simulink model "Linearization2"  (R2022a)
settings: Solver=VariableStepAuto  StartTime=0.0  StopTime=10.0  RelTol=1e-3
undefined symbols (not defined in the file): Aactuator, ac, AeroCoeff, ControlAllocation, DUmax, DUmin, EngineTable, F, fcs, ft, g, hground, IC, kg, LandingGear, Light, LPmethod, m, MIL, Mode_deflection_aileron, Mode_deflection_elevator, Mode_deflection_rudder, Mode_deflection_TVC_y, Mode_deflection_TVC_z, N, Ninv_2nozzle, Ninv_no_nozzle, PIController, s, Sensor, slug, state0, sysID_DAQ, sysID_OBES, Umax_2nozzle, Umax_no_nozzle, Umin_2nozzle, Umin_no_nozzle, WMM2020
libraries: aerolibconvert2 x19, slpidlib x6, simulink x6, sharedutil x4, aerolibatmos2 x3, aerolibwind2 x3, aerolibbdyn x3, aerolibgravity2 x2, sharedtransform x1
(part 2 of 9)

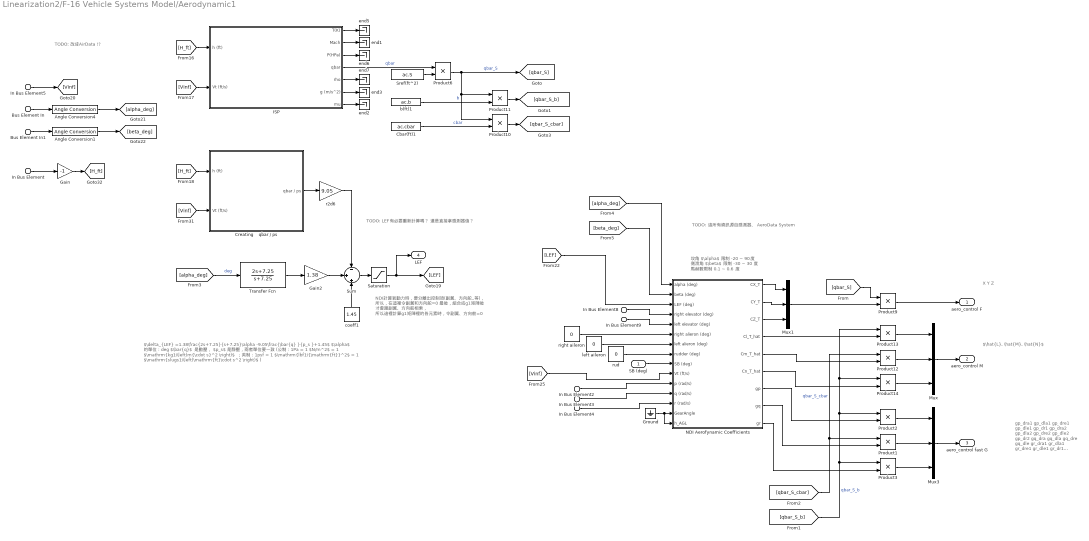
== system Linearization2/F-16 Vehicle Systems Model/Aerodynamic1 ==
  note: NDI計算氣動力時，要分離出控制項(副翼、方向舵..等)，
      | 所以，在這裡令副翼和方向舵=0
      | 最後，組合成g1矩陣後 才會跟副翼、方向舵相乘，
      | 所以這裡計算g1矩陣裡的各元素時，令副翼、方向舵=0
  note: TODO: LEF有必要重新計算嗎？
      | 還是直接拿感測器值？
  note: X
      | Y
      | Z
  note: $\delta_{LEF} =1.38\frac{2s+7.25}{s+7.25}\alpha -9.05\frac{\bar{q} }{p_s }+1.45$
      | $\alpha$ 的單位：deg
      | $\bar{q}$ 是動壓， $p_s$ 是靜壓，兩者單位要一致 (公制：1Pa = 1 $N/m^2$ = 1 $\mathrm{kg}/\left(m{\cdot s}^2 \right)$ ；英制：1psf = 1 $\mathrm{lbf}/{\mathrm{ft}}^2$ = 1 $\mathrm{slugs}/\left(\mathrm{ft}\cdot s^2 \right)$ )
  note: $\hat{L}, \hat{M}, \hat{N}$
  note: TODO: 這所有資訊源自感測器、
      | AeroData System
  note: TODO: 改成AirData !?
  note: 攻角 $\alpha$ 限制 -20 ~ 90度
      | 側滑角 $\beta$ 限制 -30 ~ 30 度
      | 馬赫數限制 0.1 ~ 0.6 度
  note: gp_dra1
      | gp_dla1
      | gp_dre1
      | gp_dle1
      | gp_dr1
      | gp_dra2
      | gp_dla2
      | gp_dre2
      | gp_dle2
      | gp_dr2
      |
      | gq_dra
      | gq_dla
      | gq_dre
      | gq_dle
      |
      | gr_dra1
      | gr_dla1
      | gr_dre1
      | gr_dle1
      | gr_dr1
      | gr_dra2
      | gr_dla2
      | gr_dre2
      | gr_dle2
      | gr_dr2
  SB (deg) : Inport  Unit=deg
  In Bus Element : Inport  Port=2  PortName=PlantData  Element=altitude
  In Bus Element8 : Inport  Port=2  PortName=PlantData  Element=AeroActBus.right Elevator_deg
  In Bus Element9 : Inport  Port=2  PortName=PlantData  Element=AeroActBus.left Elevator_deg
  In Bus Element2 : Inport  Port=2  PortName=PlantData  Element=p
  In Bus Element3 : Inport  Port=2  PortName=PlantData  Element=q
  In Bus Element4 : Inport  Port=2  PortName=PlantData  Element=r
  In Bus Element5 : Inport  Port=2  PortName=PlantData  Element=Vt
  Bus Element In : Inport  Port=3  PortName=AirData  Element=alpha
  Bus Element In1 : Inport  Port=3  PortName=AirData  Element=beta
  Angle Conversion1 : aerolibconvert2/Angle Conversion  IU=rad  OU=deg
  Angle Conversion4 : aerolibconvert2/Angle Conversion  IU=rad  OU=deg
  Cbar(ft)1 : Constant  Value=ac.cbar
  Creating    qbar / ps : Subsystem
  Gain : Gain  Gain=-1
  Gain2 : Gain  Gain=1.38  SaturateOnIntegerOverflow=on  OutDataTypeStr=Inherit: Same as input  ParamDataTypeStr=Inherit: Same as input
  Ground : Ground
  "ISP " : Subsystem
  Mux : Mux  Inputs=3
  Mux1 : Mux  Inputs=3
  Mux3 : Mux  Inputs=3
  NDI Aerofynamic Coefficients : Subsystem
  Product{1..3,6,9..14} (10 alike) : Product
  Saturation : Saturate  UpperLimit=Aactuator.LEF.AngleLimitUpper  LowerLimit=Aactuator.LEF.AngleLimitLower
  Sref(ft^2) : Constant  Value=ac.S
  Sum : Sum  Inputs=-|+|+  InputSameDT=on  SaturateOnIntegerOverflow=on  OutDataTypeStr=Inherit: Same as first input
  Transfer Fcn : TransferFcn  Numerator=[2 7.25]  Denominator=[1 7.25]
  b(ft)1 : Constant  Value=ac.b
  coeff1 : Constant  Value=1.45
  end{1..3,5..7} (6 alike) : Terminator
  left aileron : Constant  Value=0
  r2d6 : Gain  Gain=9.05  SaturateOnIntegerOverflow=on  OutDataTypeStr=Inherit: Same as input  ParamDataTypeStr=Inherit: Same as input
  right aileron : Constant  Value=0
  rud : Constant  Value=0
  aero_control F : Outport  VectorParamsAs1DForOutWhenUnconnected=off
  aero_control M : Outport  Port=2  VectorParamsAs1DForOutWhenUnconnected=off
  aero_control fast G : Outport  Port=3  VectorParamsAs1DForOutWhenUnconnected=off
  LEF : Outport  Port=4
  wires:
  [Vinf] -> "ISP "/2(Vt (ft/s))
  "ISP "/2("Mach ") -> end1/1
  "ISP "/7(mu) -> end2/1
  "ISP "/6(g (m/s^2)) -> end3/1
  "ISP "/5(rho) -> end7/1
  "ISP "/4("qbar ") -> Product6/1  "qbar"
  "ISP "/3(P(HPa)) -> end6/1
  "ISP "/1(T(K)) -> end5/1
  r2d6/1 -> Sum/1
  Creating    qbar / ps/1(qbar / ps) -> r2d6/1
  [alpha_deg] -> Transfer Fcn/1  "deg"
  [Vinf] -> Creating    qbar / ps/2(Vt (ft/s))
  coeff1/1 -> Sum/3
  [H_ft] -> Creating    qbar / ps/1(h (ft))
  [H_ft] -> "ISP "/1(h (ft))
  Sum/1 -> Saturation/1
  Saturation/1 -> LEF/1, [LEF]
  Transfer Fcn/1 -> Gain2/1
  In Bus Element/1 -> Gain/1
  Gain/1 -> [H_ft]
  Cbar(ft)1/1 -> Product10/2  "cbar"
  b(ft)1/1 -> Product11/2  "b"
  Sref(ft^2)/1 -> Product6/2
  Product10/1 -> [qbar_S_cbar]
  Product6/1 -> Product11/1, Product10/1, [qbar_S]  "qbar_S"
  Product11/1 -> [qbar_S_b]
  [qbar_S] -> Product9/1
  Product9/1 -> aero_control F/1
  Product12/1 -> Mux/2
  Product13/1 -> Mux/1
  Product14/1 -> Mux/3
  Mux/1 -> aero_control M/1
  NDI Aerofynamic Coefficients/4(Cl_T_hat) -> Product13/2
  NDI Aerofynamic Coefficients/5(Cm_T_hat) -> Product12/2
  NDI Aerofynamic Coefficients/6(Cn_T_hat) -> Product14/2
  NDI Aerofynamic Coefficients/1(CX_T) -> Mux1/1
  NDI Aerofynamic Coefficients/2(CY_T) -> Mux1/2
  NDI Aerofynamic Coefficients/3(CZ_T) -> Mux1/3
  Mux1/1 -> Product9/2
  [qbar_S_b] -> Product13/1, Product14/1, Product2/1, Product3/1  "qbar_S_b"
  Product3/1 -> Mux3/3
  Product1/1 -> Mux3/2
  Product2/1 -> Mux3/1
  NDI Aerofynamic Coefficients/7(gp) -> Product2/2
  [qbar_S_cbar] -> Product12/1, Product1/1  "qbar_S_cbar"
  NDI Aerofynamic Coefficients/9(gr) -> Product3/2
  NDI Aerofynamic Coefficients/8(gq) -> Product1/2
  Mux3/1 -> aero_control fast G/1
  [Vinf] -> NDI Aerofynamic Coefficients/10(Vt (ft/s))
  SB (deg)/1 -> NDI Aerofynamic Coefficients/9(SB (deg))
  [LEF] -> NDI Aerofynamic Coefficients/3(LEF (deg))
  [beta_deg] -> NDI Aerofynamic Coefficients/2(beta (deg))
  [alpha_deg] -> NDI Aerofynamic Coefficients/1(alpha (deg))
  In Bus Element2/1 -> NDI Aerofynamic Coefficients/11(p (rad/s))
  In Bus Element3/1 -> NDI Aerofynamic Coefficients/12(q (rad/s))
  In Bus Element4/1 -> NDI Aerofynamic Coefficients/13(r (rad/s))
  Ground/1 -> NDI Aerofynamic Coefficients/14(GearAngle), NDI Aerofynamic Coefficients/15(h_AGL)
  Gain2/1 -> Sum/2
  Bus Element In/1 -> Angle Conversion4/1
  Angle Conversion4/1 -> [alpha_deg]
  Angle Conversion1/1 -> [beta_deg]
  Bus Element In1/1 -> Angle Conversion1/1
  In Bus Element5/1 -> [Vinf]
  In Bus Element8/1 -> NDI Aerofynamic Coefficients/4(right elevator (deg))
  In Bus Element9/1 -> NDI Aerofynamic Coefficients/5(left elevator (deg))
  right aileron/1 -> NDI Aerofynamic Coefficients/6(right alieron (deg))
  left aileron/1 -> NDI Aerofynamic Coefficients/7(left alieron (deg))
  rud/1 -> NDI Aerofynamic Coefficients/8(rudder (deg))

== system Linearization2/F-16 Vehicle Systems Model/Rotation Speed(TVC OFF)OK ==
  pqr command : Inport
  In Bus Element : Inport  Port=2  PortName=PlantData  Element=Vt
  Constant : Constant  Value=0
  If : If  IfExpression=u1 > 220  ElseIfExpressions=220 >= u1 >= 135
  If Action Subsystem : Subsystem  TreatAsAtomicUnit=on
  If Action Subsystem1 : Subsystem  TreatAsAtomicUnit=on
  Merge : Merge
  Terminator1 : Terminator
  Output : Outport
  wires:
  If/1 -> If Action Subsystem/Action
  Constant/1 -> If Action Subsystem1/1(In1)
  If Action Subsystem1/1(Out1) -> Merge/2
  If Action Subsystem/1(Out1) -> Merge/1
  pqr command/1 -> If Action Subsystem/1(pqr command)
  Merge/1 -> Output/1
  In Bus Element/1 -> If/1
  If/2 -> If Action Subsystem1/Action
  If/3 -> Terminator1/1

== system Linearization2/F-16 Vehicle Systems Model/Vehicle ==
  note: 重心高度只取體軸z，因假設機腹朝下。
      | 更正確做法是要乘上旋轉座標DCM_eb
  note: 為了避免無謂計算，縮短模擬時間，
      | 只有在「飛機重心靠近地面」並且「起落架放下」的情況，
      | 才開始計算地面反作用力
  note: 設定Port dimensions=3
  note: 攻角 $\alpha$ 限制 -20 ~ 90度
      | 側滑角 $\beta$ 限制 -30 ~ 30 度
      | 馬赫數限制 0.1 ~ 0.6 度
  note: Tx
      | Ty
      | Tz
      | ---
      | Mx_T
      | My_T
      | Mz_T
  note: 高度限制 0 ~ 50000 ft
      | 馬赫數限制 0 ~ 1 馬赫
  note: f
      | 0
      | N
  note: TODO: 改成local變數
      | 或者應該新增為OBM機載模型!?
      | 或者空中NDI跟地面NDI控制器分離!?
  note: Nonlinear Model
  fadec_cmd : Inport
  fcs_cmd : Inport  Port=2
  " SB_deg" : Inport  Port=3
  LG_cmd : Inport  Port=4
  Bus Element In{,1..3} (4 alike) : Inport  Port=5  PortName=EnvData
  In Bus Element : Inport  Port=5  PortName=EnvData  Element=g
  LogDataBus : Inport  Port=6
  6DOF (Quaternion) : Subsystem
  Actuators (no roll off)1 : Subsystem  Commented=on
  Aerodynamics : Subsystem
  Bus Selector : BusSelector  OutputSignals=altitude
  Compare To Constant : simulink/Logic and Bit Operations/Compare To Constant  relop=>=  const=-30  OutDataTypeStr=boolean
  Demux2 : Demux  Outputs=[3, 3]
  Demux3 : Demux  Outputs=3
  Demux4 : Demux  Outputs=[3, 3]
  Gravity Force : Subsystem
  LandingGear GroundReaction : Subsystem
  Logical Operator : Logic  AllPortsSameDT=off  OutDataTypeStr=boolean
  Logical Operator1 : Logic  Operator=OR  Inputs=1  AllPortsSameDT=off  OutDataTypeStr=boolean
  ModelBus : BusCreator  Inputs=39
  Propulsion : Subsystem  Commented=on
  Propulsion(two_nozzles) : Subsystem
  Selector : Selector  InputPortWidth=3  IndexOptions=Index vector (dialog)  Indices=3  OutputSizes=1
  Selector1 : Selector  InputPortWidth=6  IndexOptions=Index vector (dialog)  Indices=[1 2 3]  OutputSizes=1
  Selector2 : Selector  InputPortWidth=6  IndexOptions=Index vector (dialog)  Indices=[1 2 3]  OutputSizes=1
  Signal Specification : SignalSpecification  Dimensions=3
  Sum : Sum  Inputs=||+++
  Sum1 : Sum  Inputs=++|
  Terminator3 : Terminator
  PlantData : Outport
  tag scope: LGxyz=global
  wires:
  " SB_deg"/1 -> Aerodynamics/2(" SB (deg)")
  Aerodynamics/1(FM) -> Sum/2, 6DOF (Quaternion)/4(AeroFM)
  Aerodynamics/2(ActSensor_Out) -> [AeroActBus]
  Propulsion(two_nozzles)/1(FM) -> Selector2/1, Sum/1
  fcs_cmd/1 -> Aerodynamics/1(fcs_cmd), [fcs_cmd]  "fcs_cmd"
  fadec_cmd/1 -> Propulsion(two_nozzles)/1(fadec_cmd), [fadec_cmd]  "fadec_cmd"
  Propulsion(two_nozzles)/2(ActSensor_Out) -> [PropActBus]
  Propulsion(two_nozzles)/3(PropData) -> [PropBus]
  Sum/1 -> Demux4/1
  Sum1/1 -> 6DOF (Quaternion)/1(Fxyz)
  Bus Element In/1 -> Aerodynamics/3(EnvData)
  Bus Element In1/1 -> Propulsion(two_nozzles)/2(EnvData)
  LandingGear GroundReaction/1(FM) -> Demux2/1, Sum/3, Selector1/1
  Selector1/1 -> 6DOF (Quaternion)/5(LGxyz)
  Demux2/1 -> [LGxyz]
  Demux2/2 -> Terminator3/1
  Signal Specification/1 -> Logical Operator1/1, LandingGear GroundReaction/1(LG_cmd)
  LandingGear GroundReaction/2(LGData) -> [LGBus]
  Logical Operator/1 -> LandingGear GroundReaction/Enable
  Compare To Constant/1 -> Logical Operator/1
  Bus Selector/1 -> Compare To Constant/1  "<altitude>"
  Logical Operator1/1 -> Logical Operator/2
  LG_cmd/1 -> Signal Specification/1
  Gravity Force/1(Fgrav) -> Sum1/1
  Demux4/1 -> Sum1/2
  Bus Element In3/1 -> Gravity Force/2(EnvData)
  Bus Element In2/1 -> LandingGear GroundReaction/2(EnvData)
  In Bus Element/1 -> Selector/1
  [PropActBus] -> ModelBus/35  "PropActBus"
  Demux3/2 -> ModelBus/31
  6DOF (Quaternion)/22(ay_cg) -> ModelBus/22  "ay_cg"
  Demux3/3 -> ModelBus/32  "N"
  Demux3/1 -> ModelBus/30  "f"
  6DOF (Quaternion)/2(DCM_eb) -> ModelBus/2  "DCM_eb"
  6DOF (Quaternion)/18(r) -> ModelBus/18  "r"
  6DOF (Quaternion)/8(theta) -> ModelBus/8  "theta"
  [fadec_cmd] -> ModelBus/36
  6DOF (Quaternion)/21(ax_cg) -> ModelBus/21  "ax_cg"
  [LGBus] -> ModelBus/38  "LGBus"
  6DOF (Quaternion)/3(npos) -> ModelBus/3  "npos"
  6DOF (Quaternion)/10(mu) -> ModelBus/10  "mu"
  [fcs_cmd] -> ModelBus/37
  [AeroActBus] -> ModelBus/33  "AeroActBus"
  6DOF (Quaternion)/16(p) -> ModelBus/16  "p"
  6DOF (Quaternion)/17(q) -> ModelBus/17  "q"
  6DOF (Quaternion)/13(Vt) -> ModelBus/13  "Vt"
  6DOF (Quaternion)/29(r_dot) -> ModelBus/29  "r_dot"
  6DOF (Quaternion)/24(ax_offset) -> ModelBus/24  "ax_offset"
  6DOF (Quaternion)/28(q_dot) -> ModelBus/28  "q_dot"
  6DOF (Quaternion)/19(an) -> ModelBus/19  "an"
  6DOF (Quaternion)/20(ay) -> ModelBus/20  "ay"
  6DOF (Quaternion)/6(q0q1q2q3) -> ModelBus/6  "q0q1q2q3"
  6DOF (Quaternion)/11(gamma) -> ModelBus/11  "gamma"
  6DOF (Quaternion)/27(p_dot) -> ModelBus/27  "p_dot"
  6DOF (Quaternion)/9(psi) -> ModelBus/9  "psi"
  6DOF (Quaternion)/5(altitude) -> ModelBus/5  "altitude"
  6DOF (Quaternion)/7(phi) -> ModelBus/7  "phi"
  6DOF (Quaternion)/14(alpha) -> ModelBus/14  "alpha"
  6DOF (Quaternion)/4(epos) -> ModelBus/4  "epos"
  6DOF (Quaternion)/15(beta) -> ModelBus/15  "beta"
  6DOF (Quaternion)/1(DCM_be) -> Gravity Force/1(DCM_be), ModelBus/1  "DCM_be"
  6DOF (Quaternion)/23(az_cg) -> ModelBus/23  "az_cg"
  [LGxyz] -> Demux3/1
  ModelBus/1 -> LandingGear GroundReaction/3(PlantData), Bus Selector/1, Propulsion(two_nozzles)/3(PlantData), Aerodynamics/4(PlantData), PlantData/1  "PlantData"
  6DOF (Quaternion)/25(ay_offset) -> ModelBus/25  "ay_offset"
  6DOF (Quaternion)/12(chi) -> ModelBus/12  "chi"
  [PropBus] -> ModelBus/34  "PropBus"
  6DOF (Quaternion)/26(az_offset) -> ModelBus/26  "az_offset"
  Demux4/2 -> 6DOF (Quaternion)/2(Mxyz)
  Selector2/1 -> 6DOF (Quaternion)/3(Txyz)
  Selector/1 -> 6DOF (Quaternion)/6(gravity)
  LogDataBus/1 -> ModelBus/39  "LogDataBus"

== system Linearization2/F-16 Vehicle Systems Model/pqr NDI Controller ==
  note: $\hat{L}, \hat{M}, \hat{N}$
  note: 【有向量噴嘴控制】
      | (註：有/無向量噴嘴的差異之處在於 "粉紅色模塊" 的內容)
  note: 1  gp_dra1
      |     gp_dla1
      |     gp_dre1
      |     gp_dle1
      |     gp_dr1
      |     gp_dra2
      |     gp_dla2
      |     gp_dre2
      |     gp_dle2
      |     gp_dr2
      |
      | 11 gq_dra
      |      gq_dla
      |      gq_dre
      |      gq_dle
      |
      | 15 gr_dra1
      |      gr_dla1
      |      gr_dre1
      |      gr_dle1
      |      gr_dr1
      |      gr_dra2
      |      gr_dla2
      |      gr_dre2
      |      gr_dle2
      |      gr_dr2
  note: $g_1 {\left({\overset{-}{x} }_1 \right)}={\left[\begin{array}{ccccccccc} g_{p_{\delta_{ra} } } & g_{p_{\delta_{la} } } & g_{p_{\delta_{re} } } & g_{p_{\delta_{le} } } & g_{p_{\delta_r } } & g_{p_{\delta_{ry} } } & g_{p_{\delta_{rz} } } & g_{p_{\delta_{ly} } } & g_{p_{\delta_{lz} } } \\ g_{q_{\delta_{ra} } } & g_{q_{\delta_{la} } } & g_{q_{\delta_{re} } } & g_{q_{\delta_{le} } } & 0 & g_{q_{\delta_{ry} } } & 0 & g_{q_{\delta_{ly} } } & 0 \\ g_{r_{\delta_{ra} } } & g_{r_{\delta_{la} } } & g_{r_{\delta_{re} } } & g_{r_{\delta_{le} } } & g_{r_{\delta_r } } & g_{r_{\delta_{ry} } } & g_{r_{\delta_{rz} } } & g_{r_{\delta_{ly} } } & g_{r_{\delta_{lz} } } \end{array}\right]}$
  note: 選擇偏轉模式
  coef M : Inport
  control g : Inport  Port=2
  pqr dot desire : Inport  Port=3
  p q r : Inport  Port=4
  In Bus Element : Inport  Port=5  PortName=PlantData  Element=PropBus.T
  In Bus Element12 : Inport  Port=5  PortName=PlantData  Element=alpha
  In Bus Element13 : Inport  Port=5  PortName=PlantData  Element=Vt
  In Bus Element14 : Inport  Port=5  PortName=PlantData  Element=altitude
  " f1" : MATLAB Function  TreatAsAtomicUnit=on
  Constant : Constant  Value=0
  Constant1 : Constant  Value=N
  Control Allocation : Subsystem
  Demux : Demux  Outputs=9
  Ix(slug*ft^2)1 : Constant  Value=ac.Ix
  Ixz(slug*ft^2)1 : Constant  Value=ac.Ixz
  Iy(slug*ft^2)1 : Constant  Value=ac.Iy
  Iz(slug*ft^2)1 : Constant  Value=ac.Iz
  MakeINMAT : Subsystem
  Mode_deflection : Subsystem
  Sum : Sum  Inputs=+-|
  To Workspace3 : ToWorkspace  VariableName=upast  SaveFormat=Timeseries  SampleTime=-1
  Unit Delay : UnitDelay  InitialCondition=[0 0 0 0 0 0 0 0 0]  SampleTime=fcs.Ts  HasFrameUpgradeWarning=on
  control matrix g1 : Subsystem
  left_rudder : Terminator
  "TVC_ry " : Outport  VectorParamsAs1DForOutWhenUnconnected=off
  TVC_rz : Outport  Port=2  VectorParamsAs1DForOutWhenUnconnected=off
  "TVC_ly " : Outport  Port=3  VectorParamsAs1DForOutWhenUnconnected=off
  "TVC_lz " : Outport  Port=4  VectorParamsAs1DForOutWhenUnconnected=off
  right_aileron : Outport  Port=5  VectorParamsAs1DForOutWhenUnconnected=off
  left_aileron : Outport  Port=6  VectorParamsAs1DForOutWhenUnconnected=off
  right_elevator : Outport  Port=7  VectorParamsAs1DForOutWhenUnconnected=off
  left_elevator : Outport  Port=8  VectorParamsAs1DForOutWhenUnconnected=off
  rudder : Outport  Port=9  VectorParamsAs1DForOutWhenUnconnected=off
  wires:
  coef M/1 -> " f1"/1(moments)
  p q r/1 -> " f1"/2(pqr)
  " f1"/1(f1) -> Sum/2
  pqr dot desire/1 -> Sum/1
  In Bus Element/1 -> control matrix g1/2(Thrust T)
  control g/1 -> control matrix g1/1(coef g)
  Iy(slug*ft^2)1/1 -> " f1"/4(Iy)
  Ix(slug*ft^2)1/1 -> " f1"/3(Ix)
  Iz(slug*ft^2)1/1 -> " f1"/5(Iz)
  Ixz(slug*ft^2)1/1 -> " f1"/6(Ixz)
  MakeINMAT/1(IN_MAT) -> Control Allocation/1(IN_MAT1)
  Sum/1 -> Control Allocation/5(y_bar), MakeINMAT/1(f1)
  control matrix g1/1(g1) -> MakeINMAT/2(g1), Control Allocation/6(g1)
  Control Allocation/1(Du) -> Unit Delay/1, To Workspace3/1, Demux/1
  Unit Delay/1 -> MakeINMAT/3(In3)
  In Bus Element12/1 -> Control Allocation/2(Input)
  In Bus Element13/1 -> Control Allocation/3(Input1)
  In Bus Element14/1 -> Control Allocation/4(Input2)
  Constant/1 -> Mode_deflection/6(dlr)
  Constant1/1 -> Control Allocation/7(N)
  Demux/9 -> Mode_deflection/10(dlz)
  Demux/1 -> Mode_deflection/1(dra)
  Demux/2 -> Mode_deflection/2(dla)
  Demux/5 -> Mode_deflection/5(drr)
  Demux/4 -> Mode_deflection/4(dle)
  Demux/8 -> Mode_deflection/9(dly)
  Demux/6 -> Mode_deflection/7(dry)
  Demux/3 -> Mode_deflection/3(dre)
  Demux/7 -> Mode_deflection/8(drz)
  Mode_deflection/9("TVC_ly ") -> "TVC_ly "/1
  Mode_deflection/10("TVC_lz ") -> "TVC_lz "/1
  Mode_deflection/7("TVC_ry ") -> "TVC_ry "/1
  Mode_deflection/8(TVC_rz) -> TVC_rz/1
  Mode_deflection/2(left_aileron) -> left_aileron/1
  Mode_deflection/4(left_elevator) -> left_elevator/1
  Mode_deflection/6(left_rudder) -> left_rudder/1
  Mode_deflection/1(right_aileron) -> right_aileron/1
  Mode_deflection/3(right_elevator) -> right_elevator/1
  Mode_deflection/5(rudder) -> rudder/1

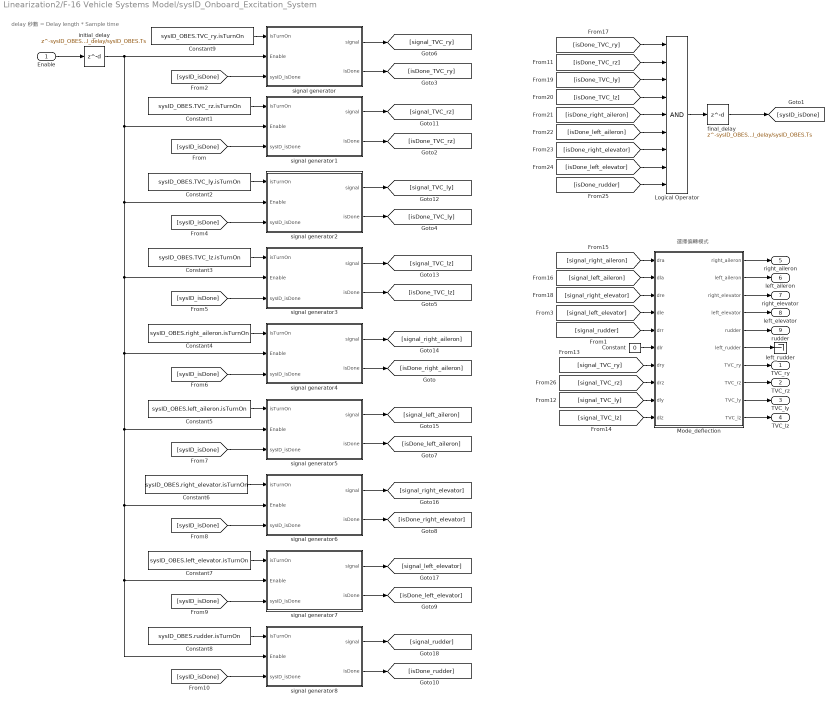
== system Linearization2/F-16 Vehicle Systems Model/sysID_Onboard_Excitation_System ==
  note: delay 秒數 = Delay length * Sample time
  note: 選擇偏轉模式
  Enable : Inport
  Constant : Constant  Value=0
  Constant1 : Constant  Value=sysID_OBES.TVC_rz.isTurnOn
  Constant2 : Constant  Value=sysID_OBES.TVC_ly.isTurnOn
  Constant3 : Constant  Value=sysID_OBES.TVC_lz.isTurnOn
  Constant4 : Constant  Value=sysID_OBES.right_aileron.isTurnOn
  Constant5 : Constant  Value=sysID_OBES.left_aileron.isTurnOn
  Constant6 : Constant  Value=sysID_OBES.right_elevator.isTurnOn
  Constant7 : Constant  Value=sysID_OBES.left_elevator.isTurnOn
  Constant8 : Constant  Value=sysID_OBES.rudder.isTurnOn
  Constant9 : Constant  Value=sysID_OBES.TVC_ry.isTurnOn
  Logical Operator : Logic  Inputs=9  AllPortsSameDT=off  OutDataTypeStr=boolean
  Mode_deflection : Subsystem
  final_delay : Delay  DelayLength=sysID_OBES.final_delay/sysID_OBES.Ts  SampleTime=sysID_OBES.Ts
  initial_delay : Delay  DelayLength=sysID_OBES.initial_delay/sysID_OBES.Ts  SampleTime=sysID_OBES.Ts
  left_rudder : Terminator
  signal generator : Subsystem  TreatAsAtomicUnit=on
  signal generator1 : Subsystem  TreatAsAtomicUnit=on
  signal generator2 : Subsystem  TreatAsAtomicUnit=on
  signal generator3 : Subsystem  TreatAsAtomicUnit=on
  signal generator4 : Subsystem  TreatAsAtomicUnit=on
  signal generator5 : Subsystem  TreatAsAtomicUnit=on
  signal generator6 : Subsystem  TreatAsAtomicUnit=on
  signal generator7 : Subsystem  TreatAsAtomicUnit=on
  signal generator8 : Subsystem  TreatAsAtomicUnit=on
  TVC_ry : Outport
  TVC_rz : Outport  Port=2
  TVC_ly : Outport  Port=3
  TVC_lz : Outport  Port=4
  right_aileron : Outport  Port=5
  left_aileron : Outport  Port=6
  right_elevator : Outport  Port=7
  left_elevator : Outport  Port=8
  rudder : Outport  Port=9
  wires:
  Logical Operator/1 -> final_delay/1
  final_delay/1 -> [sysID_isDone]
  signal generator1/2(isDone) -> [isDone_TVC_rz]
  [sysID_isDone] -> signal generator1/3(sysID_isDone)
  Enable/1 -> initial_delay/1
  signal generator/2(isDone) -> [isDone_TVC_ry]
  [sysID_isDone] -> signal generator/3(sysID_isDone)
  signal generator2/2(isDone) -> [isDone_TVC_ly]
  [sysID_isDone] -> signal generator2/3(sysID_isDone)
  signal generator3/2(isDone) -> [isDone_TVC_lz]
  [sysID_isDone] -> signal generator3/3(sysID_isDone)
  signal generator4/2(isDone) -> [isDone_right_aileron]
  [sysID_isDone] -> signal generator4/3(sysID_isDone)
  signal generator5/2(isDone) -> [isDone_left_aileron]
  [sysID_isDone] -> signal generator5/3(sysID_isDone)
  [sysID_isDone] -> signal generator6/3(sysID_isDone)
  signal generator6/2(isDone) -> [isDone_right_elevator]
  [sysID_isDone] -> signal generator7/3(sysID_isDone)
  signal generator7/2(isDone) -> [isDone_left_elevator]
  [sysID_isDone] -> signal generator8/3(sysID_isDone)
  initial_delay/1 -> signal generator1/2(Enable), signal generator2/2(Enable), signal generator3/2(Enable), signal generator4/2(Enable), signal generator5/2(Enable), signal generator6/2(Enable), signal generator8/2(Enable), signal generator7/2(Enable), signal generator/2(Enable)
  signal generator8/2(isDone) -> [isDone_rudder]
  Constant1/1 -> signal generator1/1(isTurnOn)
  Constant2/1 -> signal generator2/1(isTurnOn)
  Constant3/1 -> signal generator3/1(isTurnOn)
  Constant4/1 -> signal generator4/1(isTurnOn)
  Constant5/1 -> signal generator5/1(isTurnOn)
  Constant6/1 -> signal generator6/1(isTurnOn)
  Constant7/1 -> signal generator7/1(isTurnOn)
  Constant8/1 -> signal generator8/1(isTurnOn)
  Constant/1 -> Mode_deflection/6(dlr)
  Constant9/1 -> signal generator/1(isTurnOn)
  [isDone_TVC_ly] -> Logical Operator/3
  [isDone_TVC_lz] -> Logical Operator/4
  [isDone_right_aileron] -> Logical Operator/5
  [isDone_left_aileron] -> Logical Operator/6
  [isDone_right_elevator] -> Logical Operator/7
  [isDone_left_elevator] -> Logical Operator/8
  [signal_TVC_ry] -> Mode_deflection/7(dry)
  [isDone_rudder] -> Logical Operator/9
  [signal_TVC_ly] -> Mode_deflection/9(dly)
  [isDone_TVC_ry] -> Logical Operator/1
  [signal_TVC_lz] -> Mode_deflection/10(dlz)
  [signal_right_aileron] -> Mode_deflection/1(dra)
  [signal_left_aileron] -> Mode_deflection/2(dla)
  [signal_right_elevator] -> Mode_deflection/3(dre)
  [signal_left_elevator] -> Mode_deflection/4(dle)
  [signal_rudder] -> Mode_deflection/5(drr)
  [signal_TVC_rz] -> Mode_deflection/8(drz)
  [isDone_TVC_rz] -> Logical Operator/2
  Mode_deflection/9("TVC_ly ") -> TVC_ly/1
  Mode_deflection/10("TVC_lz ") -> TVC_lz/1
  Mode_deflection/7("TVC_ry ") -> TVC_ry/1
  Mode_deflection/8(TVC_rz) -> TVC_rz/1
  Mode_deflection/2(left_aileron) -> left_aileron/1
  Mode_deflection/4(left_elevator) -> left_elevator/1
  Mode_deflection/6(left_rudder) -> left_rudder/1
  Mode_deflection/1(right_aileron) -> right_aileron/1
  Mode_deflection/3(right_elevator) -> right_elevator/1
  Mode_deflection/5(rudder) -> rudder/1
  signal generator1/1(signal) -> [signal_TVC_rz]
  signal generator2/1(signal) -> [signal_TVC_ly]
  signal generator3/1(signal) -> [signal_TVC_lz]
  signal generator4/1(signal) -> [signal_right_aileron]
  signal generator5/1(signal) -> [signal_left_aileron]
  signal generator6/1(signal) -> [signal_right_elevator]
  signal generator7/1(signal) -> [signal_left_elevator]
  signal generator8/1(signal) -> [signal_rudder]
  signal generator/1(signal) -> [signal_TVC_ry]

== system Linearization2/F-16 Vehicle Systems Model/μαβ NDI Controller ==
  aero F : Inport
  μαβ dot desire : Inport  Port=2
  LGxyz : Inport  Port=3
  gravity : Inport  Port=4
  In Bus Element : Inport  Port=5  PortName=PlantData  Element=PropBus.T
  In Bus Element1 : Inport  Port=5  PortName=PlantData  Element=chi
  In Bus Element2 : Inport  Port=6  PortName=AirData  Element=alpha
  In Bus Element4 : Inport  Port=6  PortName=AirData  Element=alpha
  In Bus Element3 : Inport  Port=6  PortName=AirData  Element=beta
  In Bus Element5 : Inport  Port=6  PortName=AirData  Element=beta
  In Bus Element6 : Inport  Port=6  PortName=AirData  Element=mu
  In Bus Element7 : Inport  Port=6  PortName=AirData  Element=Vt
  In Bus Element8 : Inport  Port=6  PortName=AirData  Element=gamma
  Mux : Mux  Inputs=5
  Sum : Sum  Inputs=+-|
  attitude NDI : MATLAB Function  TreatAsAtomicUnit=on
  command matrix : Subsystem
  f2 : Subsystem
  pc : Outport  VectorParamsAs1DForOutWhenUnconnected=off
  qc : Outport  Port=2  VectorParamsAs1DForOutWhenUnconnected=off
  rc : Outport  Port=3  VectorParamsAs1DForOutWhenUnconnected=off
  D : Outport  Port=4  VectorParamsAs1DForOutWhenUnconnected=off
  Y : Outport  Port=5  VectorParamsAs1DForOutWhenUnconnected=off
  L : Outport  Port=6  VectorParamsAs1DForOutWhenUnconnected=off
  wires:
  f2/1(f2) -> Sum/2
  μαβ dot desire/1 -> Sum/1
  Sum/1 -> attitude NDI/1(y_bar)
  attitude NDI/1(p_c) -> pc/1
  attitude NDI/2(q_c) -> qc/1
  attitude NDI/3(r_c) -> rc/1
  command matrix/1(g2) -> attitude NDI/2(g2)
  Mux/1 -> f2/1(aero V)  "V, α, β, μ, γ"
  In Bus Element/1 -> f2/4(Thrust)
  aero F/1 -> f2/2(X,Y,Z)
  f2/2(D) -> D/1
  f2/3(Y) -> Y/1
  f2/4(L) -> L/1
  gravity/1 -> f2/3(gravity)
  In Bus Element2/1 -> command matrix/1(α)
  In Bus Element3/1 -> command matrix/2(β)
  In Bus Element5/1 -> Mux/3
  In Bus Element4/1 -> Mux/2
  In Bus Element6/1 -> Mux/4
  In Bus Element7/1 -> Mux/1
  In Bus Element8/1 -> Mux/5
  LGxyz/1 -> f2/5(LGxyz)
  In Bus Element1/1 -> f2/6(chi)

== system Linearization2/F-16 Vehicle Systems Model/Aerodynamic1/Creating    qbar // ps ==
  h (ft) : Inport
  Vt (ft/s) : Inport  Port=2
  Constant2 : Constant
  Constant3 : Constant  Value=390
  Constant6 : Constant  Value=4.14
  Math Function : Math  Operator=pow  SignedPower=on
  Math Function1 : Math  Operator=square  SignedPower=on
  Product : Product  Inputs=/*  InputSameDT=on  SaturateOnIntegerOverflow=on  OutDataTypeStr=Inherit: Same as first input
  Product5 : Product  Inputs=**  InputSameDT=on  SaturateOnIntegerOverflow=on  OutDataTypeStr=Inherit: Same as first input
  Product6 : Product  Inputs=**  InputSameDT=on  SaturateOnIntegerOverflow=on  OutDataTypeStr=Inherit: Same as first input
  Sum3 : Sum  Inputs=+-|  InputSameDT=on  SaturateOnIntegerOverflow=on  OutDataTypeStr=Inherit: Same as first input
  Switch : Switch  Threshold=35000
  r2d2 : Gain  Gain=0.703e-5  SaturateOnIntegerOverflow=on  OutDataTypeStr=Inherit: Same as input  ParamDataTypeStr=Inherit: Same as input
  r2d3 : Gain  Gain=519  SaturateOnIntegerOverflow=on  OutDataTypeStr=Inherit: Same as input  ParamDataTypeStr=Inherit: Same as input
  r2d4 : Gain  Gain=0.5  SaturateOnIntegerOverflow=on  OutDataTypeStr=Inherit: Same as input  ParamDataTypeStr=Inherit: Same as input
  r2d5 : Gain  Gain=1715  SaturateOnIntegerOverflow=on  OutDataTypeStr=Inherit: Same as input  ParamDataTypeStr=Inherit: Same as input
  rho0 : Gain  Gain=2.377e-3  SaturateOnIntegerOverflow=on  OutDataTypeStr=Inherit: Same as input  ParamDataTypeStr=Inherit: Same as input
  qbar / ps : Outport  VectorParamsAs1DForOutWhenUnconnected=off
  wires:
  h (ft)/1 -> r2d2/1, Switch/2
  Sum3/1 -> Math Function/1, r2d3/1  "tfac"
  Constant3/1 -> Switch/1
  r2d3/1 -> Switch/3
  Constant6/1 -> Math Function/2
  rho0/1 -> Product5/1, Product6/2  "rho"
  r2d2/1 -> Sum3/2
  Constant2/1 -> Sum3/1
  Math Function/1 -> rho0/1
  Math Function1/1 -> Product5/2
  Switch/1 -> r2d5/1  "temp"
  r2d5/1 -> Product6/1
  Product6/1 -> Product/1  "ps"
  Product5/1 -> r2d4/1  "qbar"
  Product/1 -> qbar / ps/1
  Vt (ft/s)/1 -> Math Function1/1  "Vt (ft/s)"
  r2d4/1 -> Product/2

== system Linearization2/F-16 Vehicle Systems Model/Aerodynamic1/ISP  ==
  note: 1 T
      | 2 a (Speed of sound)
      | 3 P
      | 4 rho
      | 5 g
      | 6 mu (Coefficient of viscosity)
  h (ft) : Inport
  Vt (ft/s) : Inport  Port=2
  Demux : Demux  Outputs=[1,1,1,1,1,1]
      settings: DisplayOption=none
  Divide1 : Product  Inputs=*/
  Length Conversion : aerolibconvert2/Length Conversion  IU=ft  OU=m
  MATLAB Function : MATLAB Function  TreatAsAtomicUnit=on
  Product : Product
  Square : Math  Operator=square  SignedPower=on
  To Workspace : ToWorkspace  VariableName=mach  SaveFormat=Timeseries  SampleTime=-1
  r2d1 : Gain  Gain=0.5  SaturateOnIntegerOverflow=on  OutDataTypeStr=Inherit: Same as input  ParamDataTypeStr=Inherit: Same as input
  r2d3 : Gain  Gain=3.2808399  SaturateOnIntegerOverflow=on  OutDataTypeStr=Inherit: Same as input  ParamDataTypeStr=Inherit: Same as input
  r2d4 : Gain  Gain=0.00194032033  SaturateOnIntegerOverflow=on  OutDataTypeStr=Inherit: Same as input  ParamDataTypeStr=Inherit: Same as input
  T(K) : Outport  VectorParamsAs1DForOutWhenUnconnected=off
  "Mach " : Outport  Port=2  VectorParamsAs1DForOutWhenUnconnected=off
  P(HPa) : Outport  Port=3  VectorParamsAs1DForOutWhenUnconnected=off
  "qbar " : Outport  Port=4  VectorParamsAs1DForOutWhenUnconnected=off
  rho : Outport  Port=5  VectorParamsAs1DForOutWhenUnconnected=off
  g (m/s^2) : Outport  Port=6  VectorParamsAs1DForOutWhenUnconnected=off
  mu : Outport  Port=7  VectorParamsAs1DForOutWhenUnconnected=off
  wires:
  r2d3/1 -> Divide1/2
  r2d1/1 -> Product/2
  Demux/4 -> rho/1, r2d4/1  "rho(kg/m^3)"
  Demux/2 -> r2d3/1  "a(m/s)"
  Demux/1 -> T(K)/1  "T(K)"
  r2d4/1 -> r2d1/1
  Divide1/1 -> To Workspace/1, "Mach "/1
  Demux/5 -> g (m/s^2)/1  "g (m/s^2)"
  Demux/6 -> mu/1  "mu"
  Product/1 -> "qbar "/1
  Square/1 -> Product/1
  Vt (ft/s)/1 -> Square/1, Divide1/1
  Demux/3 -> P(HPa)/1  "P(Pa)"
  h (ft)/1 -> Length Conversion/1
  Length Conversion/1 -> MATLAB Function/1(h)
  MATLAB Function/1(ISP_output) -> Demux/1

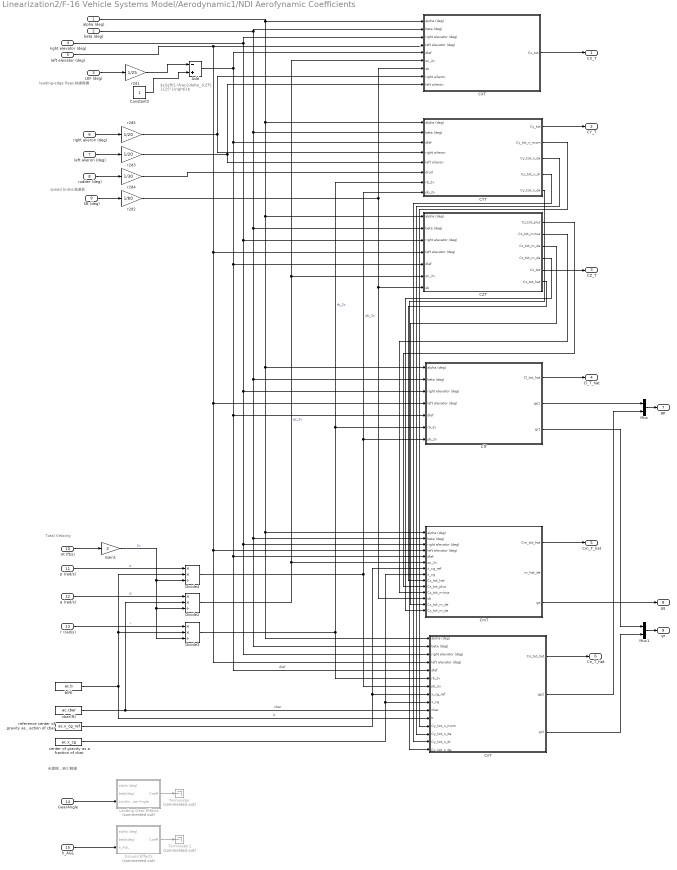
== system Linearization2/F-16 Vehicle Systems Model/Aerodynamic1/NDI Aerofynamic Coefficients ==
  note: leading-edge flaps
      | 前緣襟翼
  note: speed brake
      | 減速板
  note: Total Velocity
  note: 未建模，缺少數據
  note: ${\left(1-\frac{\delta_{LEF} }{25°}\right)}$
  alpha (deg) : Inport
  beta (deg) : Inport  Port=2
  LEF (deg) : Inport  Port=3
  right elevator (deg) : Inport  Port=4
  left elevator (deg) : Inport  Port=5
  right alieron (deg) : Inport  Port=6
  left alieron (deg) : Inport  Port=7
  rudder (deg) : Inport  Port=8
  SB (deg) : Inport  Port=9  Unit=deg
  Vt (ft/s) : Inport  Port=10
  p (rad/s) : Inport  Port=11
  q (rad/s) : Inport  Port=12
  r (rad/s) : Inport  Port=13
  GearAngle : Inport  Port=14
  h_AGL : Inport  Port=15
  Add : Sum  Inputs=-+
  CXT : Subsystem
  CYT : Subsystem
  CZT : Subsystem
  ClT : Subsystem
  CmT : Subsystem
  CnT : Subsystem
  Constant3 : Constant
  Divide2 : Product  Inputs=**/
  Divide3 : Product  Inputs=**/
  Divide4 : Product  Inputs=**/
  Gain1 : Gain  Gain=2
  Ground Effects : Subsystem  Commented=on
  Landing Gear Effects : Subsystem  Commented=on
  Mux : Mux  Inputs=2
  Mux1 : Mux  Inputs=2
  Terminator : Terminator  Commented=on
  Terminator1 : Terminator  Commented=on
  b(ft) : Constant  Value=ac.b
  cbar(ft) : Constant  Value=ac.cbar
  center of gravity as a fraction of cbar : Constant  Value=ac.x_cg
  r2d1 : Gain  Gain=1/25  SaturateOnIntegerOverflow=on  OutDataTypeStr=Inherit: Same as input  ParamDataTypeStr=Inherit: Same as input
  r2d2 : Gain  Gain=1/60  SaturateOnIntegerOverflow=on  OutDataTypeStr=Inherit: Same as input  ParamDataTypeStr=Inherit: Same as input
  r2d3 : Gain  Gain=1/20  SaturateOnIntegerOverflow=on  OutDataTypeStr=Inherit: Same as input  ParamDataTypeStr=Inherit: Same as input
  r2d4 : Gain  Gain=1/30  SaturateOnIntegerOverflow=on  OutDataTypeStr=Inherit: Same as input  ParamDataTypeStr=Inherit: Same as input
  r2d5 : Gain  Gain=1/20  SaturateOnIntegerOverflow=on  OutDataTypeStr=Inherit: Same as input  ParamDataTypeStr=Inherit: Same as input
  reference center of gravity as a fraction of cbar : Constant  Value=ac.x_cg_ref
  CX_T : Outport  VectorParamsAs1DForOutWhenUnconnected=off
  CY_T : Outport  Port=2  VectorParamsAs1DForOutWhenUnconnected=off
  CZ_T : Outport  Port=3  VectorParamsAs1DForOutWhenUnconnected=off
  Cl_T_hat : Outport  Port=4  VectorParamsAs1DForOutWhenUnconnected=off
  Cm_T_hat : Outport  Port=5  VectorParamsAs1DForOutWhenUnconnected=off
  Cn_T_hat : Outport  Port=6  VectorParamsAs1DForOutWhenUnconnected=off
  gp : Outport  Port=7  VectorParamsAs1DForOutWhenUnconnected=off
  gq : Outport  Port=8  VectorParamsAs1DForOutWhenUnconnected=off
  gr : Outport  Port=9  VectorParamsAs1DForOutWhenUnconnected=off
  wires:
  alpha (deg)/1 -> CXT/1(alpha (deg)), CnT/1(alpha (deg)), CmT/1(alpha (deg)), ClT/1(alpha (deg)), CZT/1(alpha (deg)), CYT/1(alpha (deg))
  beta (deg)/1 -> CXT/2(beta (deg)), CnT/2(beta (deg)), CmT/2(beta (deg)), ClT/2(beta (deg)), CZT/2(beta (deg)), CYT/2(beta (deg))
  right elevator (deg)/1 -> CXT/3(right elevator (deg)), CnT/3(right elevator (deg)), CmT/3(right elevator (deg)), ClT/3(right elevator (deg)), CZT/3(right elevator (deg))
  Vt (ft/s)/1 -> Gain1/1
  p (rad/s)/1 -> Divide4/1  "p"
  q (rad/s)/1 -> Divide2/1  "q"
  r (rad/s)/1 -> Divide3/1  "r"
  b(ft)/1 -> Divide4/2, Divide3/2, CnT/11(b)  "b"
  cbar(ft)/1 -> Divide2/2, CnT/10(cbar)  "cbar"
  Add/1 -> CXT/5(dlef), CnT/5(dlef), CmT/5(dlef), ClT/5(dlef), CZT/5(dlef), CYT/3(dlef)  "dlef"
  left alieron (deg)/1 -> r2d3/1
  rudder (deg)/1 -> r2d4/1
  Divide2/1 -> CXT/6(qc_2v), CZT/6(qc_2v), CmT/6(qc_2v)  "qc_2v"
  r2d4/1 -> CYT/6(drud)
  Divide3/1 -> CnT/6(rb_2v), CYT/7(rb_2v), ClT/6(rb_2v)  "rb_2v"
  Divide4/1 -> CnT/7(pb_2v), CYT/8(pb_2v), ClT/7(pb_2v)  "pb_2v"
  reference center of gravity as a fraction of cbar/1 -> CmT/7(x_cg_ref), CnT/8(x_cg_ref)
  center of gravity as a fraction of cbar/1 -> CmT/8(x_cg), CnT/9(x_cg)
  CZT/1(Cz_tot_plus) -> CmT/10(Cz_tot_plus)
  CZT/2(Cz_tot_minus) -> CmT/11(Cz_tot_minus)
  CYT/2(Cy_tot_n_mom) -> CnT/12(Cy_tot_n_mom)
  CYT/3(Cy_tot_n_da) -> CnT/13(Cy_tot_n_da)
  CYT/4(Cy_tot_n_dr) -> CnT/14(Cy_tot_n_dr)
  SB (deg)/1 -> r2d2/1
  CXT/1(Cx_tot) -> CX_T/1
  CYT/1(Cy_tot) -> CY_T/1
  CZT/5(Cz_tot) -> CZ_T/1
  CnT/1(Cn_tot_hat) -> Cn_T_hat/1
  CmT/1(Cm_tot_hat) -> Cm_T_hat/1
  ClT/1(Cl_tot_hat) -> Cl_T_hat/1
  LEF (deg)/1 -> r2d1/1
  r2d2/1 -> CXT/7(sb), CmT/12(sb), CZT/7(sb)
  Gain1/1 -> Divide3/3, Divide2/3, Divide4/3  "2v"
  Landing Gear Effects/1(Coeff) -> Terminator/1
  h_AGL/1 -> Ground Effects/3(h_AGL)
  Ground Effects/1(Coeff) -> Terminator1/1
  GearAngle/1 -> Landing Gear Effects/3(Landing Gear Angle)
  right alieron (deg)/1 -> r2d5/1
  r2d5/1 -> CXT/8(right aileron), CYT/4(right aileron)
  r2d3/1 -> CYT/5(left aileron), CXT/9(left aileron)
  r2d1/1 -> Add/1
  Constant3/1 -> Add/2
  left elevator (deg)/1 -> CXT/4(left elevator (deg)), CnT/4(left elevator (deg)), CmT/4(left elevator (deg)), ClT/4(left elevator (deg)), CZT/4(left elevator (deg))
  Mux1/1 -> gr/1
  CmT/3(gq) -> gq/1
  CnT/3(gr2) -> Mux1/2
  ClT/3(gr1) -> Mux1/1
  CnT/2(gp2) -> Mux/2
  Mux/1 -> gp/1
  ClT/2(gp1) -> Mux/1
  CZT/6(Cz_tot_hat) -> CmT/9(Cz_tot_hat)
  CYT/5(Cy_tot_n_de) -> CnT/15(Cy_tot_n_de)
  CZT/3(Cz_tot_m_de) -> CmT/13(Cz_tot_m_de)
  CZT/4(Cz_tot_m_da) -> CmT/14(Cz_tot_m_da)

== system Linearization2/F-16 Vehicle Systems Model/Rotation Speed(TVC OFF)OK/If Action Subsystem ==
  pqr command : Inport
  Action Port : ActionPort  ActionPortLabel=if( u1 > 220)
  Out1 : Outport
  wires:
  pqr command/1 -> Out1/1

== system Linearization2/F-16 Vehicle Systems Model/Rotation Speed(TVC OFF)OK/If Action Subsystem1 ==
  In1 : Inport
  Action Port : ActionPort  ActionPortLabel=elseif(220 >= u1 >= 135)
  Mux1 : Mux  Inputs=3
  Out1 : Outport
  wires:
  In1/1 -> Mux1/3, Mux1/1, Mux1/2
  Mux1/1 -> Out1/1  "pqr dot desire"

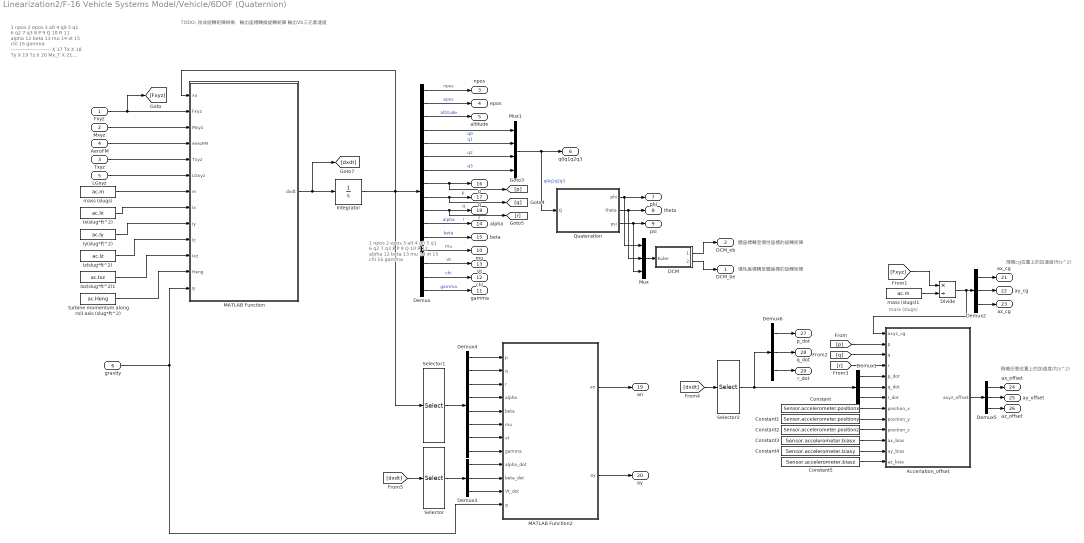
== system Linearization2/F-16 Vehicle Systems Model/Vehicle/6DOF (Quaternion) ==
  note: TODO: 改成旋轉矩陣相乘、輸出座標轉換旋轉矩陣
      | 輸出Vb三元素速度
  note: 1 npos
      | 2 epos
      | 3 alt
      | 4 q0
      | 5 q1
      | 6 q2
      | 7 q3
      | 8 P
      | 9 Q
      | 10 R
      | 11 alpha
      | 12 beta
      | 13 mu
      | 14 vt
      | 15 chi
      | 16 gamma
      | ------------------------
      | X 17 Tx
      | X 18 Ty
      | X 19 Tz
      | X 20 Mx_T
      | X 21 My_T
      | X 22 Mz_T
      | X 23 T
      | --------------------
      | X 24 ele
      | X 25 ail
      | X 26 rud
      | -------------------
      | X 27 delta_z
      | X 28 delta_y
      | -----------------
      | X 29 qbar
      | -----------------
      | X 30 CXT
      | X 31 CYT
      | X 32 CZT
      | X 33 CLT
      | X 34 CMT
      | X 35 CNT
      | -----------------
      | X 36 lef
  note: 1 npos
      | 2 epos
      | 3 alt
      | 4 q0
      | 5 q1
      | 6 q2
      | 7 q3
      | 8 P
      | 9 Q
      | 10 R
      | 11 alpha
      | 12 beta
      | 13 mu
      | 14 vt
      | 15 chi
      | 16 gamma
  note: 慣性座標轉至體座標的旋轉矩陣
  note: 體座標轉至慣性座標的旋轉矩陣
  note: mass (slugs)
  note: 飛機cg位置上的加速度(ft/s^2)
  note: 飛機任意位置上的加速度(ft/s^2)
  Fxyz : Inport
  Mxyz : Inport  Port=2
  Txyz : Inport  Port=3
  AeroFM : Inport  Port=4
  LGxyz : Inport  Port=5
  gravity : Inport  Port=6
  Accerlation_offset : Subsystem
  Constant : Constant  Value=Sensor.accelerometer.positionx
  Constant1 : Constant  Value=Sensor.accelerometer.positiony
  Constant2 : Constant  Value=Sensor.accelerometer.positionz
  Constant3 : Constant  Value=Sensor.accelerometer.biasx
  Constant4 : Constant  Value=Sensor.accelerometer.biasy
  Constant5 : Constant  Value=Sensor.accelerometer.biasz
  DCM : Subsystem
  Demux : Demux  Outputs=16
      settings: DisplayOption=none
  Demux{1..3,5..6} (5 alike) : Demux  Outputs=3
  Demux4 : Demux  Outputs=8
  Divide : Product  Inputs=*/
  Integrator : Integrator  InitialCondition=state0  ContinuousStateAttributes={'npos', 'epos', 'alt', 'q0', 'q1', 'q2', 'q3', 'P', 'Q', 'R', 'alpha', 'beta', 'mu', 'vt', 'chi', 'gamma'}
  Ix(slug*ft^2) : Constant  Value=ac.Ix
  Ixz(slug*ft^2)1 : Constant  Value=ac.Ixz
  Iy(slug*ft^2) : Constant  Value=ac.Iy
  Iz(slug*ft^2) : Constant  Value=ac.Iz
  MATLAB Function : MATLAB Function  TreatAsAtomicUnit=on
  MATLAB Function2 : MATLAB Function  TreatAsAtomicUnit=on
  Mux : Mux  Inputs=3
  Mux1 : Mux  Inputs=[1,1,1,1]
  Quateration : MATLAB Function  TreatAsAtomicUnit=on
  Selector : Selector  InputPortWidth=16  IndexOptions=Index vector (dialog)  Indices=[11 12 14]  OutputSizes=3
  Selector1 : Selector  InputPortWidth=16  IndexOptions=Index vector (dialog)  Indices=[8:14 16]  OutputSizes=3
  Selector2 : Selector  InputPortWidth=16  IndexOptions=Index vector (dialog)  Indices=[8 9 10]  OutputSizes=3
  mass (slugs) : Constant  Value=ac.m
  mass (slugs)1 : Constant  Value=ac.m
  turbine momentum along roll axis (slug*ft^2) : Constant  Value=ac.Heng
  DCM_be : Outport
  DCM_eb : Outport  Port=2
  npos : Outport  Port=3  VectorParamsAs1DForOutWhenUnconnected=off
  epos : Outport  Port=4  VectorParamsAs1DForOutWhenUnconnected=off
  altitude : Outport  Port=5  VectorParamsAs1DForOutWhenUnconnected=off
  q0q1q2q3 : Outport  Port=6
  phi : Outport  Port=7  VectorParamsAs1DForOutWhenUnconnected=off
  theta : Outport  Port=8  VectorParamsAs1DForOutWhenUnconnected=off
  psi : Outport  Port=9  VectorParamsAs1DForOutWhenUnconnected=off
  mu : Outport  Port=10  VectorParamsAs1DForOutWhenUnconnected=off
  gamma : Outport  Port=11  VectorParamsAs1DForOutWhenUnconnected=off
  chi : Outport  Port=12  VectorParamsAs1DForOutWhenUnconnected=off
  Vt : Outport  Port=13  VectorParamsAs1DForOutWhenUnconnected=off
  alpha : Outport  Port=14  VectorParamsAs1DForOutWhenUnconnected=off
  beta : Outport  Port=15  VectorParamsAs1DForOutWhenUnconnected=off
  p : Outport  Port=16  VectorParamsAs1DForOutWhenUnconnected=off
  q : Outport  Port=17  VectorParamsAs1DForOutWhenUnconnected=off
  r : Outport  Port=18  VectorParamsAs1DForOutWhenUnconnected=off
  an : Outport  Port=19
  ay : Outport  Port=20
  ax_cg : Outport  Port=21
  ay_cg : Outport  Port=22
  az_cg : Outport  Port=23
  ax_offset : Outport  Port=24
  ay_offset : Outport  Port=25
  az_offset : Outport  Port=26
  p_dot : Outport  Port=27
  q_dot : Outport  Port=28
  r_dot : Outport  Port=29
  wires:
  Demux/2 -> epos/1  "epos"
  Demux/3 -> altitude/1  "altitude"
  Integrator/1 -> MATLAB Function/1(xu), Demux/1, Selector1/1
  Demux/1 -> npos/1  "npos"
  Demux/5 -> Mux1/2  "q1"
  Demux/4 -> Mux1/1  "q0"
  Demux/7 -> Mux1/4  "q3"
  Demux/6 -> Mux1/3  "q2"
  Demux/8 -> p/1, [p]  "p"
  Demux/9 -> q/1, [q]  "q"
  Demux/10 -> r/1, [r]  "r"
  Demux/11 -> alpha/1  "alpha"
  Demux/12 -> beta/1  "beta"
  Demux/13 -> mu/1  "mu"
  Demux/14 -> Vt/1  "Vt"
  Demux/15 -> chi/1  "chi"
  Demux/16 -> gamma/1  "gamma"
  Mux1/1 -> q0q1q2q3/1, Quateration/1(Q)  "q0q1q2q3"
  AeroFM/1 -> MATLAB Function/4(AeroFM)
  Mxyz/1 -> MATLAB Function/3(Mxyz)
  Fxyz/1 -> [Fxyz], MATLAB Function/2(Fxyz)
  Txyz/1 -> MATLAB Function/5(Txyz)
  gravity/1 -> MATLAB Function2/12(g), MATLAB Function/13(g)
  Ix(slug*ft^2)/1 -> MATLAB Function/8(Ix)
  Iy(slug*ft^2)/1 -> MATLAB Function/9(Iy)
  Iz(slug*ft^2)/1 -> MATLAB Function/10(Iz)
  Ixz(slug*ft^2)1/1 -> MATLAB Function/11(Ixz)
  turbine momentum along roll axis (slug*ft^2)/1 -> MATLAB Function/12(Heng)
  mass (slugs)/1 -> MATLAB Function/7(m)
  Selector/1 -> Demux3/1
  Demux3/1 -> MATLAB Function2/9(alpha_dot)
  Demux3/2 -> MATLAB Function2/10(beta_dot)
  Demux3/3 -> MATLAB Function2/11(Vt_dot)
  Selector1/1 -> Demux4/1
  Demux4/1 -> MATLAB Function2/1(p)
  Demux4/2 -> MATLAB Function2/2(q)
  Demux4/3 -> MATLAB Function2/3(r)
  Demux4/4 -> MATLAB Function2/4(alpha)
  Demux4/5 -> MATLAB Function2/5(beta)
  Demux4/6 -> MATLAB Function2/6(mu)
  Demux4/7 -> MATLAB Function2/7(vt)
  Demux4/8 -> MATLAB Function2/8(gamma)
  MATLAB Function2/1(an) -> an/1
  MATLAB Function2/2(ay) -> ay/1
  LGxyz/1 -> MATLAB Function/6(LGxyz)
  Quateration/3(psi) -> Mux/3, psi/1
  Quateration/2(theta) -> theta/1, Mux/2
  Quateration/1(phi) -> phi/1, Mux/1
  Mux/1 -> DCM/1(Euler)
  DCM/1(DCM_eb) -> DCM_eb/1
  DCM/2(DCM_be) -> DCM_be/1
  Constant4/1 -> Accerlation_offset/12(ay_bias)
  Accerlation_offset/1(axyz_offset) -> Demux5/1
  Constant/1 -> Accerlation_offset/8(position_x)
  Selector2/1 -> Demux6/1, Demux1/1
  Demux6/1 -> p_dot/1
  Demux1/2 -> Accerlation_offset/6(q_dot)
  Demux6/2 -> q_dot/1
  Demux5/1 -> ax_offset/1
  Demux5/3 -> az_offset/1
  Demux6/3 -> r_dot/1
  [dxdt] -> Selector2/1
  Demux2/1 -> ax_cg/1
  mass (slugs)1/1 -> Divide/2
  Demux1/1 -> Accerlation_offset/5(p_dot)
  Demux1/3 -> Accerlation_offset/7(r_dot)
  [p] -> Accerlation_offset/2(p)
  [Fxyz] -> Divide/1
  [q] -> Accerlation_offset/3(q)
  Constant1/1 -> Accerlation_offset/9(position_y)
  [r] -> Accerlation_offset/4(r)
  Constant3/1 -> Accerlation_offset/11(ax_bias)
  Constant5/1 -> Accerlation_offset/13(az_bias)
  Demux2/3 -> az_cg/1
  Divide/1 -> Accerlation_offset/1(axyz_cg), Demux2/1
  Constant2/1 -> Accerlation_offset/10(position_z)
  Demux5/2 -> ay_offset/1
  Demux2/2 -> ay_cg/1
  MATLAB Function/1(dxdt) -> [dxdt], Integrator/1
  [dxdt] -> Selector/1

== system Linearization2/F-16 Vehicle Systems Model/Vehicle/Actuators (no roll off)1 ==
  note: 這種建模方式會得到跟順淵不同的結果
  Command : Inport
  "Mach " : Inport  Port=2
  alt : Inport  Port=3
  alpha,beta : Inport  Port=4
  Aileron Saturation : Saturate  UpperLimit=21.5  LowerLimit=-21.5
  Demux1 : Demux  Outputs=6
  Elevator Saturation : Saturate  UpperLimit=25  LowerLimit=-25
  Engine block : Subsystem
  Fcn : Fcn  Expr=u(1)*cos(u(2))*cos(u(3))
  Integrator (degrees) : Integrator  Commented=through  InitialCondition=0.015206  UpperSaturationLimit=30  LowerSaturationLimit=-30
  Integrator (degrees)1 : Integrator  Commented=through  UpperSaturationLimit=30  LowerSaturationLimit=-30
  Integrator (degrees)2 : Integrator  Commented=on  UpperSaturationLimit=30  LowerSaturationLimit=-30
  Integrator(degrees) : Integrator  Commented=on  InitialCondition=-0.051516  UpperSaturationLimit=21.5  LowerSaturationLimit=-21.5
  "Integrator(degrees) " : Integrator  Commented=on  InitialCondition=-4.2454  UpperSaturationLimit=25  LowerSaturationLimit=-25
  Mux1 : Mux  Inputs=2
  Mux9 : Mux  Inputs=6
  Rate Limiter : RateLimiter  RisingSlewLimit=+60  FallingSlewLimit=-60  SampleTimeMode=inherited
  Rate Limiter1 : RateLimiter  RisingSlewLimit=+80  FallingSlewLimit=-80  SampleTimeMode=inherited
  Rate Limiter2 : RateLimiter  RisingSlewLimit=+120  FallingSlewLimit=-120  SampleTimeMode=inherited
  Rate Limiter3 : RateLimiter  RisingSlewLimit=+60  FallingSlewLimit=-60  SampleTimeMode=inherited
  Rate Limiter4 : RateLimiter  RisingSlewLimit=+60  FallingSlewLimit=-60  SampleTimeMode=inherited
  Rudder Saturation : Saturate  UpperLimit=30  LowerLimit=-30
  Saturation : Saturate  UpperLimit=50000  LowerLimit=0
  Saturation Dynamic : simulink/Discontinuities/Saturation Dynamic  OutMin=[]  OutMax=[]  OutDataTypeStr=Inherit: Same as second input  OutDataType=fixdt(1, 16)  OutScaling=2^-10  DoSatur=off
  TVC_Y Saturation : Saturate  UpperLimit=15  LowerLimit=-15
  TVC_Z Saturation : Saturate  UpperLimit=15  LowerLimit=-15
  Transfer Fcn{,1..4} (5 alike) : TransferFcn  Numerator=[20.202]  Denominator=[1 20.202]
  r2d2 : Gain  Gain=-1  SaturateOnIntegerOverflow=on  OutDataTypeStr=Inherit: Same as input  ParamDataTypeStr=Inherit: Same as input
  Actuator : Outport  VectorParamsAs1DForOutWhenUnconnected=off
  wires:
  Mux9/1 -> Actuator/1
  Command/1 -> Demux1/1
  Transfer Fcn/1 -> Mux9/2  "elevator"
  Transfer Fcn1/1 -> Mux9/3  "Aileron"
  Transfer Fcn2/1 -> Mux9/4  "Rudder"
  Saturation Dynamic/1 -> Mux9/1  "thrust"
  Transfer Fcn4/1 -> Mux9/6  "yaw vector"
  Transfer Fcn3/1 -> Mux9/5  "pitch vector"
  r2d2/1 -> Saturation/1
  alt/1 -> r2d2/1
  Demux1/1 -> Saturation Dynamic/2
  "Mach "/1 -> Mux1/1
  alpha,beta/1 -> Mux1/2
  Mux1/1 -> Fcn/1
  Fcn/1 -> Engine block/1(Mach)
  Saturation/1 -> Engine block/2(Attitude)
  Engine block/2(T_min) -> Saturation Dynamic/3
  Engine block/1(T_max) -> Saturation Dynamic/1
  Demux1/2 -> Elevator Saturation/1
  Elevator Saturation/1 -> Rate Limiter/1
  Demux1/3 -> Aileron Saturation/1
  Aileron Saturation/1 -> Rate Limiter1/1
  Demux1/4 -> Rudder Saturation/1
  Rudder Saturation/1 -> Rate Limiter2/1
  Demux1/5 -> TVC_Z Saturation/1
  TVC_Z Saturation/1 -> Rate Limiter3/1
  Demux1/6 -> TVC_Y Saturation/1
  TVC_Y Saturation/1 -> Rate Limiter4/1
  Rate Limiter/1 -> Transfer Fcn/1
  Rate Limiter1/1 -> Transfer Fcn1/1
  Rate Limiter2/1 -> Transfer Fcn2/1
  Rate Limiter3/1 -> Transfer Fcn3/1
  Rate Limiter4/1 -> Transfer Fcn4/1
